simulink model "practica5simu"  (R2026a)
settings: Solver=ode45  StopTime=0.005
settings Model: Creator=themi  LastModifiedBy=themi

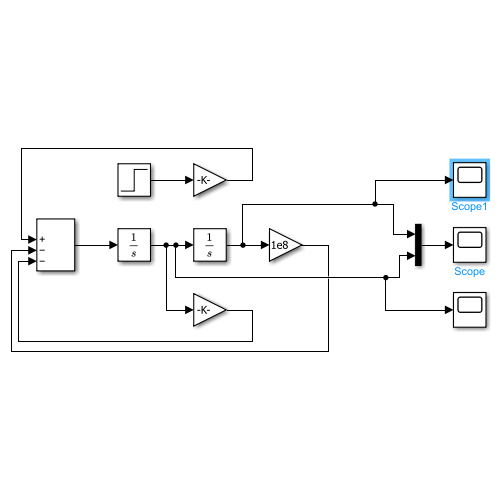
[thumbnail: Simulink's stored preview of the top-level diagram]
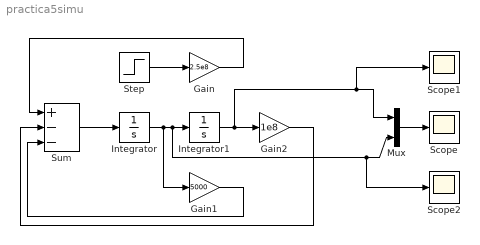
== system practica5simu ==
  Gain : Gain  Gain=2.5e8
  Gain1 : Gain  Gain=5000
  Gain2 : Gain  Gain=1e8
  Integrator : Integrator
  Integrator1 : Integrator  InitialCondition=1
  Mux : Mux  Inputs=2
  Scope : Scope
      settings: ActiveDisplayYMinimum=-8233.1991531881  ActiveDisplayYMaximum=13046.443166728393
  Scope1 : Scope
      settings: ActiveDisplayYMinimum=0.730775960318188  ActiveDisplayYMaximum=3.4230163571363081
  Scope2 : Scope
      settings: ActiveDisplayYMinimum=-1  ActiveDisplayYMaximum=1  DataLoggingVariableName=ScopeData2
  Step : Step  Time=0  SampleTime=0
  Sum : Sum  Inputs=|+--
  wires:
  Step/1 -> Gain/1
  Integrator/1 -> Gain1/1, Scope2/1, Mux/2, Integrator1/1
  Integrator1/1 -> Scope1/1, Mux/1, Gain2/1
  Gain/1 -> Sum/1
  Sum/1 -> Integrator/1
  Gain2/1 -> Sum/2
  Gain1/1 -> Sum/3
  Mux/1 -> Scope/1
